simulink model "ACC_Project"  (R2022a)
settings: Solver=FixedStepDiscrete  StartTime=0.0  StopTime=10.0  FixedStep=0.01  MaxStep=0.01  RelTol=1e-3
settings Model: DataDictionary=Adaptive_Cruise_Control.sldd  Creator=Rohan More  LastModifiedBy=Rohan More
settings OptimizationCC: DefaultParameterBehavior=Inlined  EnhancedBackFolding=on  PassReuseOutputArgsAs=Individual arguments  ZeroExternalMemoryAtStartup=off  ZeroInternalMemoryAtStartup=off  OptimizeBlockOrder=speed  DifferentSizesBufferReuse=on  OptimizationCustomize=off  EfficientTunableParamExpr=on
settings DebuggingCC: ParameterTunabilityLossMsg=error
settings SFSimCC: MATLABDynamicMemAlloc=off
settings RTWCC: SystemTargetFile=ert.tlc  TemplateMakefile=ert_default_tmf
settings CodeAppCC: ForceParamTrailComments=on  IgnoreCustomStorageClasses=off  OperatorAnnotations=on  SimulinkDataObjDesc=on  SFDataObjDesc=on  InsertBlockDesc=on
settings ERTTargetCC: TargetLangStandard=C99 (ISO)  GenerateSampleERTMain=on  InlinedParameterPlacement=NonHierarchical  ERTCustomFileTemplate=example_file_process.tlc

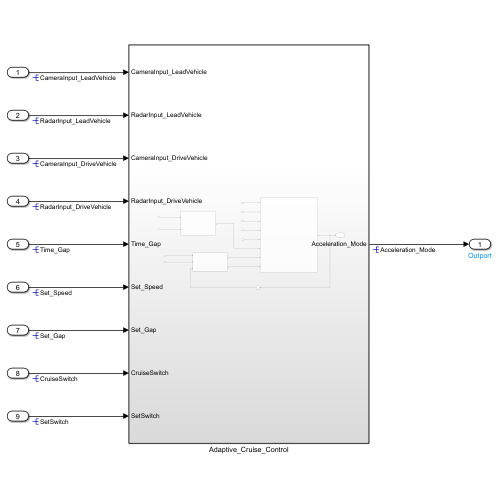
[thumbnail: Simulink's stored preview of the top-level diagram]
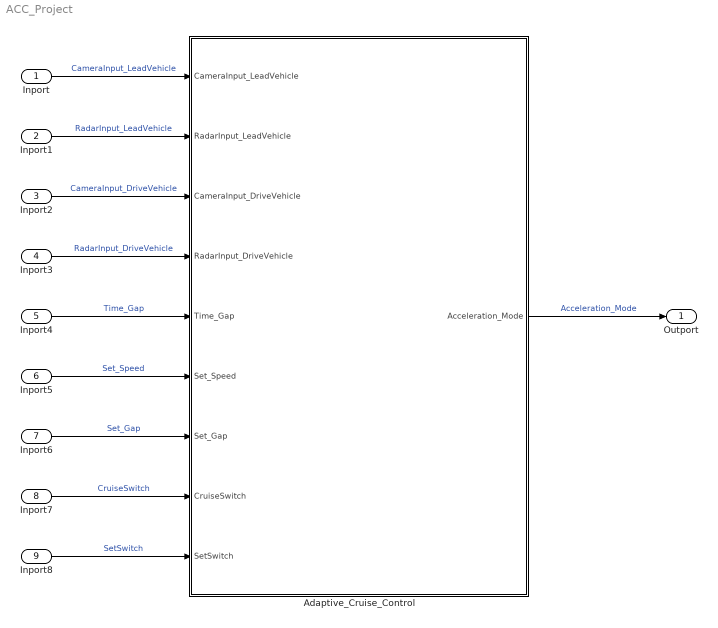
== system ACC_Project ==
  Inport : Inport
  Inport1 : Inport  Port=2
  Inport2 : Inport  Port=3
  Inport3 : Inport  Port=4
  Inport4 : Inport  Port=5
  Inport5 : Inport  Port=6
  Inport6 : Inport  Port=7
  Inport7 : Inport  Port=8
  Inport8 : Inport  Port=9
  Adaptive_Cruise_Control : Subsystem
  Outport : Outport
  wires:
  Inport/1 -> Adaptive_Cruise_Control/1(CameraInput_LeadVehicle)  "CameraInput_LeadVehicle"
  Inport1/1 -> Adaptive_Cruise_Control/2(RadarInput_LeadVehicle)  "RadarInput_LeadVehicle"
  Inport2/1 -> Adaptive_Cruise_Control/3(CameraInput_DriveVehicle)  "CameraInput_DriveVehicle"
  Inport3/1 -> Adaptive_Cruise_Control/4(RadarInput_DriveVehicle)  "RadarInput_DriveVehicle"
  Inport4/1 -> Adaptive_Cruise_Control/5(Time_Gap)  "Time_Gap"
  Inport5/1 -> Adaptive_Cruise_Control/6(Set_Speed)  "Set_Speed"
  Inport6/1 -> Adaptive_Cruise_Control/7(Set_Gap)  "Set_Gap"
  Inport7/1 -> Adaptive_Cruise_Control/8(CruiseSwitch)  "CruiseSwitch"
  Inport8/1 -> Adaptive_Cruise_Control/9(SetSwitch)  "SetSwitch"
  Adaptive_Cruise_Control/1(Acceleration_Mode) -> Outport/1  "Acceleration_Mode"

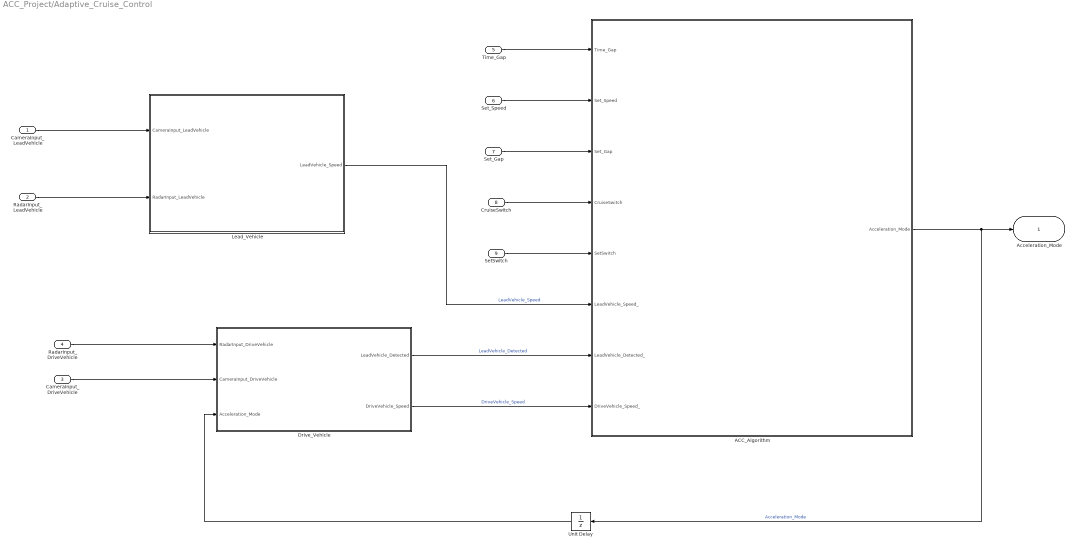
== system ACC_Project/Adaptive_Cruise_Control ==
  CameraInput_LeadVehicle : Inport
  RadarInput_LeadVehicle : Inport  Port=2
  CameraInput_DriveVehicle : Inport  Port=3
  RadarInput_DriveVehicle : Inport  Port=4
  Time_Gap : Inport  Port=5
  Set_Speed : Inport  Port=6
  Set_Gap : Inport  Port=7
  CruiseSwitch : Inport  Port=8
  SetSwitch : Inport  Port=9
  ACC_Algorithm : Subsystem
  Drive_Vehicle : Subsystem
  Lead_Vehicle : Subsystem
  Unit Delay : UnitDelay  SampleTime=-1  HasFrameUpgradeWarning=on
  Acceleration_Mode : Outport
  wires:
  CameraInput_LeadVehicle/1 -> Lead_Vehicle/1(CameraInput_LeadVehicle)
  RadarInput_LeadVehicle/1 -> Lead_Vehicle/2(RadarInput_LeadVehicle)
  Lead_Vehicle/1(LeadVehicle_Speed) -> ACC_Algorithm/6(LeadVehicle_Speed_)  "LeadVehicle_Speed"
  Time_Gap/1 -> ACC_Algorithm/1(Time_Gap)
  Set_Speed/1 -> ACC_Algorithm/2(Set_Speed)
  Set_Gap/1 -> ACC_Algorithm/3(Set_Gap)
  CruiseSwitch/1 -> ACC_Algorithm/4(CruiseSwitch)
  SetSwitch/1 -> ACC_Algorithm/5(SetSwitch)
  ACC_Algorithm/1(Acceleration_Mode) -> Unit Delay/1, Acceleration_Mode/1  "Acceleration_Mode"
  RadarInput_DriveVehicle/1 -> Drive_Vehicle/1(RadarInput_DriveVehicle)
  CameraInput_DriveVehicle/1 -> Drive_Vehicle/2(CameraInput_DriveVehicle)
  Drive_Vehicle/1(LeadVehicle_Detected) -> ACC_Algorithm/7(LeadVehicle_Detected_)  "LeadVehicle_Detected"
  Drive_Vehicle/2(DriveVehicle_Speed) -> ACC_Algorithm/8(DriveVehicle_Speed_)  "DriveVehicle_Speed"
  Unit Delay/1 -> Drive_Vehicle/3(Acceleration_Mode)

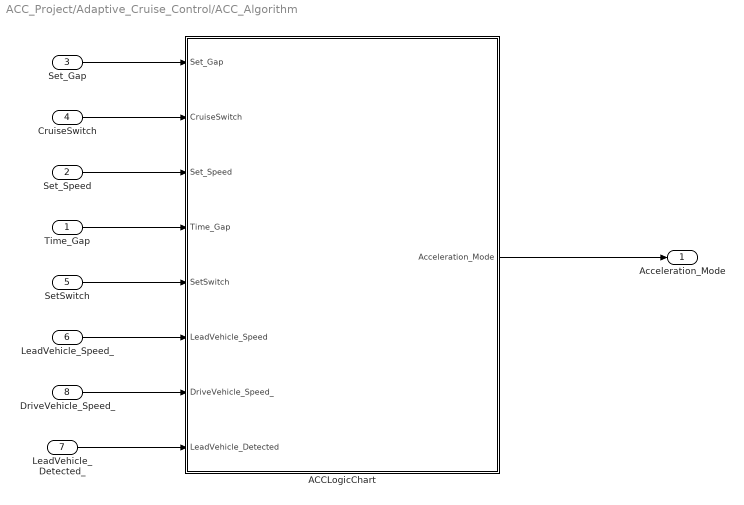
== system ACC_Project/Adaptive_Cruise_Control/ACC_Algorithm ==
  Time_Gap : Inport
  Set_Speed : Inport  Port=2
  Set_Gap : Inport  Port=3
  CruiseSwitch : Inport  Port=4
  SetSwitch : Inport  Port=5
  LeadVehicle_Speed_ : Inport  Port=6
  LeadVehicle_Detected_ : Inport  Port=7
  DriveVehicle_Speed_ : Inport  Port=8
  ACCLogicChart : Stateflow chart  TreatAsAtomicUnit=on
  Acceleration_Mode : Outport
  wires:
  LeadVehicle_Detected_/1 -> ACCLogicChart/8(LeadVehicle_Detected)
  Set_Gap/1 -> ACCLogicChart/1(Set_Gap)
  Time_Gap/1 -> ACCLogicChart/4(Time_Gap)
  DriveVehicle_Speed_/1 -> ACCLogicChart/7(DriveVehicle_Speed_)
  LeadVehicle_Speed_/1 -> ACCLogicChart/6(LeadVehicle_Speed)
  Set_Speed/1 -> ACCLogicChart/3(Set_Speed)
  SetSwitch/1 -> ACCLogicChart/5(SetSwitch)
  CruiseSwitch/1 -> ACCLogicChart/2(CruiseSwitch)
  ACCLogicChart/1(Acceleration_Mode) -> Acceleration_Mode/1

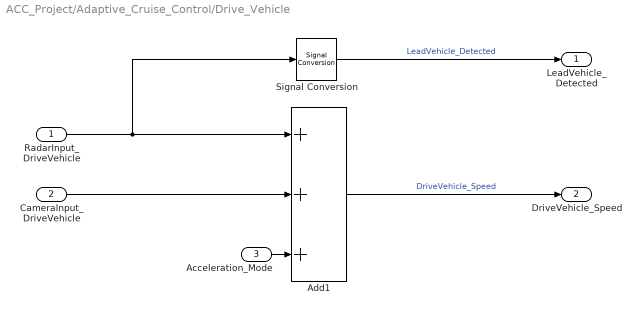
== system ACC_Project/Adaptive_Cruise_Control/Drive_Vehicle ==
  RadarInput_DriveVehicle : Inport
  CameraInput_DriveVehicle : Inport  Port=2
  Acceleration_Mode : Inport  Port=3
  Add1 : Sum  Inputs=+++
  Signal Conversion : SignalConversion  OverrideOpt=off
  LeadVehicle_Detected : Outport
  DriveVehicle_Speed : Outport  Port=2
  wires:
  Acceleration_Mode/1 -> Add1/3
  RadarInput_DriveVehicle/1 -> Signal Conversion/1, Add1/1
  CameraInput_DriveVehicle/1 -> Add1/2
  Add1/1 -> DriveVehicle_Speed/1  "DriveVehicle_Speed"
  Signal Conversion/1 -> LeadVehicle_Detected/1  "LeadVehicle_Detected"

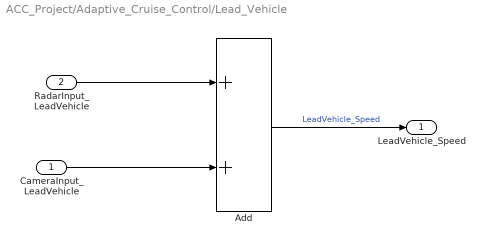
== system ACC_Project/Adaptive_Cruise_Control/Lead_Vehicle ==
  CameraInput_LeadVehicle : Inport
  RadarInput_LeadVehicle : Inport  Port=2
  Add : Sum
  LeadVehicle_Speed : Outport
  wires:
  Add/1 -> LeadVehicle_Speed/1  "LeadVehicle_Speed"
  CameraInput_LeadVehicle/1 -> Add/2
  RadarInput_LeadVehicle/1 -> Add/1

== stateflow chart ACC_Project/Adaptive_Cruise_Control/ACC_Algorithm/ACCLogicChart ==
  state ACC_OFF_MODE
    entry:
    Acceleration_Mode = 0;
  state ACC_STANDBY_MODE
    entry:
    Acceleration_Mode = 1;
  state ACC_ON_MODE
    state LeadVehicle_Not_Detected_Resume
      entry:
      Acceleration_Mode = 1;
    state LeadVehicle_Detected_Follow
      entry:
      Acceleration_Mode =2;
    state LeadVehicle_Detected_Resume
      entry:
      Acceleration_Mode =3;
    state LeadVehicle_Not_Detected
      entry:
      Acceleration_Mode = 1;
    state LeadVehicle_Speed_equal_Set_Speed
      entry:
      Acceleration_Mode = 5;
    state LeadVehicle_Speed_lessthan_Set_Speed
      entry:
      Acceleration_Mode = 4;
    (default) -> LeadVehicle_Detected_Follow
    LeadVehicle_Detected_Resume -> LeadVehicle_Not_Detected_Resume [order 1] : [LeadVehicle_Detected == 0]
    LeadVehicle_Detected_Resume -> LeadVehicle_Detected_Follow [order 3] : [(DriveVehicle_Speed == Set_Speed) && ...
        | (LeadVehicle_Speed >= Set_Speed) && ...
        | (Time_Gap >= Set_Gap)]
    LeadVehicle_Detected_Follow -> LeadVehicle_Not_Detected [order 2] : [LeadVehicleDetected == 0]
    LeadVehicle_Not_Detected -> LeadVehicle_Detected_Follow [order 2] : [(LeadVehicle_Detected == 1) && ...
        | (DriveVehicle_Speed == Set_Speed) && ...
        |  (LeadVehicle_Speed >= Set_Speed) && ...
        | (Time_Gap >= Set_Gap)]
    LeadVehicle_Speed_equal_Set_Speed -> LeadVehicle_Detected_Resume [order 2] : [(DriveVehicle_Speed < Set_Speed) && ...
        | (LeadVehicle_Speed > DriveVehicle_Speed) ||...
        | (Time_Gap >= Set_Gap)]
    LeadVehicle_Detected_Resume -> LeadVehicle_Speed_equal_Set_Speed [order 2] : [(LeadVehicle_Speed*1.25 >= DriveVehicle_Speed) && ...
        | (LeadVehicle_Speed*0.75 <= DriveVehicle_Speed) && ...
        | (DriveVehicle_Speed < Set_Speed) && ...
        | (Time_Gap <= 1.25*Set_Gap) && ...
        | (Time_Gap >= 0.75*Set_Gap)]
    LeadVehicle_Speed_equal_Set_Speed -> LeadVehicle_Not_Detected_Resume [order 1] : [(LeadVehicle_Detected == 0) || ...
        | (DriveVehicle_Speed <= Set_Speed)]
    LeadVehicle_Detected_Follow -> LeadVehicle_Speed_lessthan_Set_Speed [order 1] : [(LeadVehicle_Detected == 1) && ...
        | (LeadVehicle_Speed < Set_Speed) || ...
        | (Time_Gap < Set_Gap)]
    LeadVehicle_Speed_lessthan_Set_Speed -> LeadVehicle_Not_Detected [order 1] : [(LeadVehicle_Detected == 0) && ...
        | (DriveVehicle_Speed == Set_Speed)]
    LeadVehicle_Not_Detected -> LeadVehicle_Speed_lessthan_Set_Speed [order 1] : [(LeadVehicle_Detected == 1) && ...
        | (LeadVehicle_Speed < Set_Speed) || ...
        | (Time_Gap < Set_Gap)]
    LeadVehicle_Speed_equal_Set_Speed -> LeadVehicle_Speed_lessthan_Set_Speed [order 3] : [(LeadVehicle_Speed < Set_Speed) && ...
        | (LeadVehicle_Speed < DriveVehicle_Speed) || ...
        | (Time_Gap == 0.75*Set_Gap)]
    LeadVehicle_Speed_lessthan_Set_Speed -> LeadVehicle_Speed_equal_Set_Speed [order 2] : [(LeadVehicle_Speed*1.25 >= DriveVehicle_Speed) && ...
        | (LeadVehicle_Speed*0.75 <= DriveVehicle_Speed) && ...
        | (DriveVehicle_Speed < Set_Speed) && ...
        | (Time_Gap <= 1.25*Set_Gap) && ...
        | (Time_Gap >= 0.75*Set_Gap)]
  (default) -> ACC_OFF_MODE
  ACC_STANDBY_MODE -> ACC_OFF_MODE [order 2] : [CruiseSwitch == 0]
  ACC_OFF_MODE -> ACC_STANDBY_MODE : [CruiseSwitch == 1]
  ACC_ON_MODE -> ACC_OFF_MODE [order 2] : [CruiseSwitch == 0]
  ACC_STANDBY_MODE -> ACC_ON_MODE [order 1] : [SetSwitch == 1]
  ACC_ON_MODE -> ACC_STANDBY_MODE [order 1] : [SetSwitch == 0]
  data: Set_Gap input; CruiseSwitch input; Set_Speed input; Time_Gap input; SetSwitch input; Acceleration_Mode output; LeadVehicle_Speed input; DriveVehicle_Speed_ input; LeadVehicle_Detected input
